simulink model "BiCopter_CBF"  (R2024a)
settings: Solver=ode4  StartTime=0.0  StopTime=100  FixedStep=0.005  RelTol=1e-3
values from neighbouring files (symbols this model uses):
  k = lqr(A,B,Q,R)    [K_Mat.m]
libraries: simulink_extras x2, shared6dof x1
settings Model: Creator=moham  LastModifiedBy=sepehrmahfar
settings OptimizationCC: ReuseModelBlockBuffer=off
settings RTWCC: GPUComputeCapability=3.5

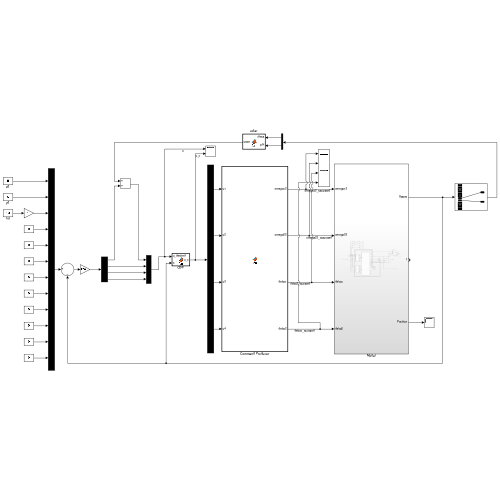
[thumbnail: Simulink's stored preview of the top-level diagram]
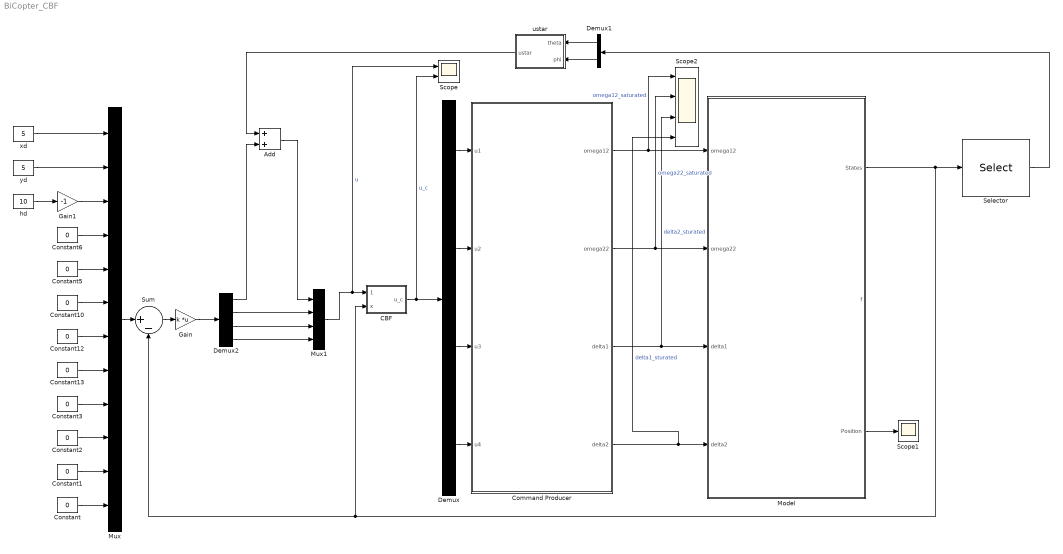
== system BiCopter_CBF ==
  Add : Sum
  CBF : MATLAB Function  TreatAsAtomicUnit=on
  Command Producer : MATLAB Function  TreatAsAtomicUnit=on
  Constant{,1..3,5..6,10,12..13} (9 alike) : Constant  Value=0
  Demux : Demux
  Demux1 : Demux  Outputs=2
  Demux2 : Demux
  Gain : Gain  Gain=k  Multiplication=Matrix(K*u)
  Gain1 : Gain  Gain=-1
  Model : Subsystem
  Mux : Mux  Inputs=12
  Mux1 : Mux
  Scope : Scope  NumInputPorts=2
  Scope1 : Scope
  Scope2 : Scope  NumInputPorts=4
  Selector : Selector  InputPortWidth=12  IndexOptions=Index vector (dialog)  Indices=[7 8]  OutputSizes=1
  Sum : Sum  Inputs=|+-
  hd : Constant  Value=10
  ustar : MATLAB Function  TreatAsAtomicUnit=on
  xd : Constant  Value=5
  yd : Constant  Value=5
  wires:
  Constant/1 -> Mux/12
  Model/1(States) -> Selector/1, CBF/2(x), Sum/2
  Mux/1 -> Sum/1
  Constant1/1 -> Mux/11
  Constant2/1 -> Mux/10
  hd/1 -> Gain1/1
  Constant6/1 -> Mux/4
  Constant5/1 -> Mux/5
  Constant10/1 -> Mux/6
  Gain1/1 -> Mux/3
  Command Producer/4(delta2) -> Scope2/4, Model/4(delta2)  "delta1_sturated"
  Command Producer/3(delta1) -> Scope2/3, Model/3(delta1)  "delta2_sturated"
  Command Producer/2(omega22) -> Scope2/2, Model/2(omega22)  "omega22_saturated"
  Command Producer/1(omega12) -> Scope2/1, Model/1(omega12)  "omega12_saturated"
  Demux/4 -> Command Producer/4(u4)
  Demux/3 -> Command Producer/3(u3)
  Demux/2 -> Command Producer/2(u2)
  ustar/1(ustar) -> Add/1
  Constant12/1 -> Mux/7
  Constant13/1 -> Mux/8
  Sum/1 -> Gain/1
  CBF/1(u_c) -> Demux/1, Scope/2  "u_c"
  Gain/1 -> Demux2/1
  Demux2/1 -> Add/2
  Add/1 -> Mux1/1
  Demux2/2 -> Mux1/2
  Demux2/3 -> Mux1/3
  Demux2/4 -> Mux1/4
  Mux1/1 -> Scope/1, CBF/1(u_desired)  "u"
  Demux/1 -> Command Producer/1(u1)
  xd/1 -> Mux/1
  yd/1 -> Mux/2
  Selector/1 -> Demux1/1
  Demux1/2 -> ustar/2(phi)
  Demux1/1 -> ustar/1(theta)
  Model/3(Position) -> Scope1/1
  Constant3/1 -> Mux/9

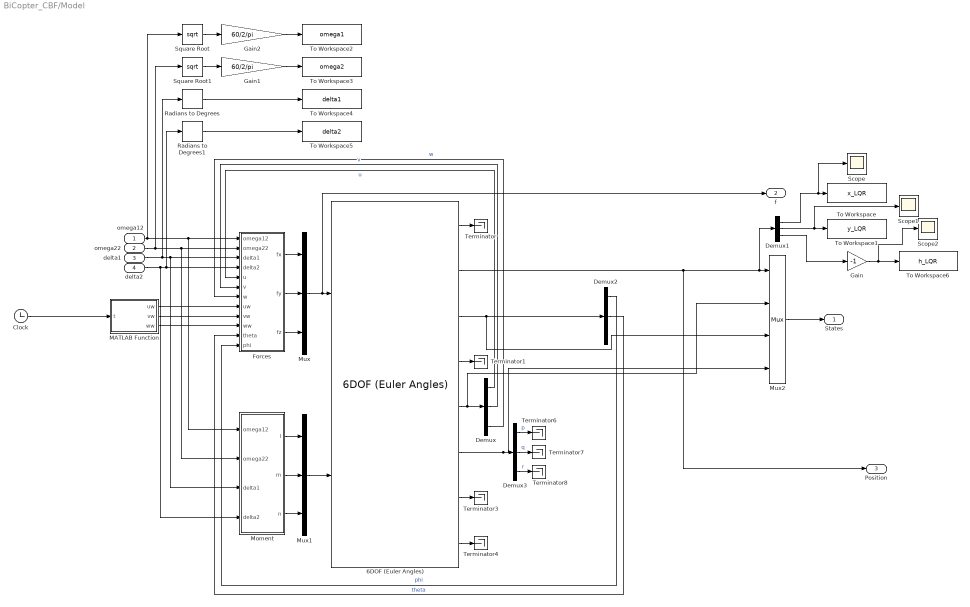
== system BiCopter_CBF/Model ==
  omega12 : Inport
  omega22 : Inport  Port=2
  delta1 : Inport  Port=3
  delta2 : Inport  Port=4
  6DOF (Euler Angles) : shared6dof/6DOF (Euler Angles)  units=Metric (MKS)  mtype=Fixed  rep=Euler Angles  xme_0=[2 0 0]  Vm_0=[0 0 0]  eul_0=[0 0 0]  pm_0=[0 0 0]  mass_0=0.296  mass_e=0.5  mass_f=2.0  inertia=[0.0049, 0, -0.003675; 0, 0.0049, 0; -0.003675, 0, 0.0088]  inertia_e=eye(3)  inertia_f=2*eye(3)  k_quat=1.0  vre_flag=on  abi_flag=off  aMode=0  xme_statename=''  Vm_statename=''  eul_statename=''  quat_statename=''  pm_statename=''  mass_statename=''
  Clock : Clock
  Demux{,1..3} (4 alike) : Demux  Outputs=3
  Forces : MATLAB Function  TreatAsAtomicUnit=on
  Gain : Gain  Gain=-1
  Gain1 : Gain  Gain=60/2/pi
  Gain2 : Gain  Gain=60/2/pi
  MATLAB Function : MATLAB Function  TreatAsAtomicUnit=on
  Moment : MATLAB Function  TreatAsAtomicUnit=on
  Mux : Mux  Inputs=3
  Mux1 : Mux  Inputs=3
  Mux2 : Mux
  Radians to Degrees : simulink_extras/Transformations/Radians to Degrees
  Radians to Degrees1 : simulink_extras/Transformations/Radians to Degrees
  Scope : Scope
  Scope1 : Scope
  Scope2 : Scope
  Square Root : Sqrt
  Square Root1 : Sqrt
  Terminator{,1,3..4,6..8} (7 alike) : Terminator
  To Workspace : ToWorkspace  VariableName=x_LQR  SampleTime=-1
      settings: Save2DSignal=2-D array (concatenate along first dimension)
  To Workspace1 : ToWorkspace  VariableName=y_LQR  SampleTime=-1
      settings: Save2DSignal=2-D array (concatenate along first dimension)
  To Workspace2 : ToWorkspace  VariableName=omega1  SampleTime=-1
      settings: Save2DSignal=2-D array (concatenate along first dimension)
  To Workspace3 : ToWorkspace  VariableName=omega2  SampleTime=-1
      settings: Save2DSignal=2-D array (concatenate along first dimension)
  To Workspace4 : ToWorkspace  VariableName=delta1  SampleTime=-1
      settings: Save2DSignal=2-D array (concatenate along first dimension)
  To Workspace5 : ToWorkspace  VariableName=delta2  SampleTime=-1
      settings: Save2DSignal=2-D array (concatenate along first dimension)
  To Workspace6 : ToWorkspace  VariableName=h_LQR  SampleTime=-1
      settings: Save2DSignal=2-D array (concatenate along first dimension)
  States : Outport
  f : Outport  Port=2
  Position : Outport  Port=3
  wires:
  Moment/1(l) -> Mux1/1
  delta1/1 -> Moment/3(delta1), Forces/3(delta1), Radians to Degrees/1
  6DOF (Euler Angles)/5 -> Mux2/2, Demux/1
  Demux2/2 -> Forces/11(theta)  "theta"
  Mux/1 -> f/1, 6DOF (Euler Angles)/1
  6DOF (Euler Angles)/2 -> Position/1, Demux1/1, Mux2/1
  Forces/1(fx) -> Mux/1
  Forces/2(fy) -> Mux/2
  Mux1/1 -> 6DOF (Euler Angles)/2
  6DOF (Euler Angles)/4 -> Terminator1/1
  Demux/1 -> Forces/5(u)  "u"
  Clock/1 -> MATLAB Function/1(t)
  Demux2/1 -> Forces/12(phi)  "phi"
  Demux/2 -> Forces/6(v)  "v"
  omega12/1 -> Moment/1(omega12), Forces/1(omega12), Square Root/1
  6DOF (Euler Angles)/8 -> Terminator4/1
  6DOF (Euler Angles)/1 -> Terminator/1
  Moment/3(n) -> Mux1/3
  6DOF (Euler Angles)/7 -> Terminator3/1
  Moment/2(m) -> Mux1/2
  Forces/3(fz) -> Mux/3
  Demux/3 -> Forces/7(w)  "w"
  6DOF (Euler Angles)/3 -> Mux2/3, Demux2/1
  6DOF (Euler Angles)/6 -> Mux2/4, Demux3/1
  omega22/1 -> Moment/2(omega22), Forces/2(omega22), Square Root1/1
  delta2/1 -> Radians to Degrees1/1, Forces/4(delta2), Moment/4(delta2)
  Demux3/1 -> Terminator6/1  "p"
  Demux3/2 -> Terminator7/1  "q"
  Demux3/3 -> Terminator8/1  "r"
  Mux2/1 -> States/1
  Demux1/2 -> Scope1/1, To Workspace1/1
  Demux1/1 -> Scope/1, To Workspace/1
  Square Root/1 -> Gain2/1
  Square Root1/1 -> Gain1/1
  Radians to Degrees/1 -> To Workspace4/1
  Radians to Degrees1/1 -> To Workspace5/1
  Demux1/3 -> Gain/1
  Gain/1 -> Scope2/1, To Workspace6/1
  Gain1/1 -> To Workspace3/1
  Gain2/1 -> To Workspace2/1
  MATLAB Function/3(ww) -> Forces/10(ww)
  MATLAB Function/2(vw) -> Forces/9(vw)
  MATLAB Function/1(uw) -> Forces/8(uw)

== matlab function BiCopter_CBF/Model/Moment ==
  data: omega12 input; omega22 input; delta1 input; delta2 input; l output; m output; n output
function [l, m, n] = fcn(omega12, omega22, delta1, delta2)
a = 0.225;
h = 0.0225;
b = 2.98e-6;
d = 1.14e-7;
l = a*b*(omega12*cos(delta1)-omega22*cos(delta2)) + d*(-omega12*sin(delta1)+omega22*sin(delta2));
m = -b*h*(omega12*sin(delta1)+omega22*sin(delta2));
n = a*b*(omega12*sin(delta1)-omega22*sin(delta2)) + d*(omega12*cos(delta1)-omega22*cos(delta2));

== matlab function BiCopter_CBF/Model/Forces ==
  data: omega12 input; omega22 input; delta1 input; delta2 input; u input; fx output; v input; w input; uw input; vw input; ww input; theta input; phi input; fy output; fz output
function [fx, fy, fz] = fcn(omega12, omega22, delta1, delta2, u, v, w, uw, vw, ww, theta, phi)
ua = u - uw;
va = v - vw;
wa = w - ww;
m = 0.296;
g = 9.81;
rho = 1.2682;
s = 0.25;
CD = 0.32;
b = 2.98e-6;
fx = -m*g*sin(theta) - 0.5*rho*s*CD*sqrt(ua^2+va^2+wa^2)*ua + b*(omega12*sin(delta1)+omega22*sin(delta2));
fy = m*g*sin(phi)*cos(theta) - 0.5*rho*s*CD*sqrt(ua^2+va^2+wa^2)*va;
fz = m*g*cos(phi)*cos(theta) - 0.5*rho*s*CD*sqrt(ua^2+va^2+wa^2)*wa - b*(omega12*cos(delta1)+omega22*cos(delta2));

== matlab function BiCopter_CBF/Command Producer ==
  data: u1 input; omega12 output; omega22 output; delta1 output; delta2 output; u2 input; u3 input; u4 input
function [omega12, omega22, delta1, delta2] = fcn(u1, u2, u3, u4)
delta1 = atan2((u3+u4), (u1+u2));
delta2 = atan2((u3-u4), (u1-u2));
omega12 = 0.5 * (u1+u2) / cos(delta1);
omega22 = 0.5 * (u1-u2) / cos(delta2);
% a = 0.225;
% h = 0.0225;
% b = 2.98e-6;
% d = 1.14e-7;
% delta1 = atan2(b*h*(d*u2-b*a*u4) + ((d^2)+((b^2)*(a^2))*u3), b*h*(d*u4+b*a*u2) - h*(d^2)+((b^2)*(a^2))*u1);
% delta2 = atan2(b*h*(d*u2-b*a*u4) - ((d^2)+((b^2)*(a^2))*u3), b*h*(d*u4+b*a*u2) + h*(d^2)+((b^2)*(a^2))*u1);
% omega12 = ((b*h*(d*u2-b*a*u4) + ((d^2)+((b^2)*(a^2))*u3))^2) + (h^2)*((b*(d*u4 + b*a*u2) - ((d^2)+(b^2)*(a^2))*u1)^2) / (2*b*h*((d^2)+(b^2)*(a^2)));
% omega22 = ((b*h*(d*u2-b*a*u4) - ((d^2)+((b^2)*(a^2))*u3))^2) + (h^2)*((b*(d*u4 + b*a*u2) + ((d^2)+(b^2)*(a^2))*u1)^2) / (2*b*h*((d^2)+(b^2)*(a^2)));

== matlab function BiCopter_CBF/Model/MATLAB Function ==
  data: t input; uw output; vw output; ww output
function [uw, vw, ww] = fcn(t)
uw = 0;
vw = 0;
ww = 0;

== matlab function BiCopter_CBF/ustar ==
  data: theta input; phi input; ustar output
function ustar  = fcn(theta, phi)
g = 9.81;
b = 2.98e-6;
m = 0.296;
ustar = m * g / b * cos(theta) * cos(phi);

== matlab function BiCopter_CBF/CBF ==
  data: u_desired input; u_c output; x input
function u_c = fcn(u_desired, x)
z_min = -7;
m = 0.296;
g = 9.81;
rho = 1.2682;
s = 0.25;
b = 2.98e-6;
CD = 0.32;
h =  x(3) - z_min;
alpha = 0.3;
dz_dx = [0, 0, 1, 0, 0, 0, 0, 0, 0, 0, 0, 0];
F = [0
    0
    -x(4)*sin(x(8))+x(5)*(sin(x(7))*cos(x(8)))+x(6)*cos(x(7))*cos(x(8))
    0
    0
    0
    0
    0
    0
    0
    0
    0];
g_aff = zeros(12,4);
H = 2*eye(4);
f = -2*u_desired;
A = -dz_dx *g_aff;
b = alpha*h+dz_dx*F;
options = optimoptions('quadprog','Algorithm','active-set');
[u_c, ~, ~, ~] = quadprog(H, f, A, b, [], [], [], [], zeros(4,1), options);


end
